simulink model "CAMFC2_Quad_New_02_Payload_01"  (R2018b)
settings: Solver=ode45  StartTime=0.0  StopTime=200  RelTol=1e-3  EnableMultiTasking=on
InitFcn:
  | constant_CAMFC2_Quad_New_02_Payload_01
values from neighbouring files (symbols this model uses):
  alpha = 0.01    [constant_CAMFC2_Quad_New_02_Payload_01.m]
  AN = [     0 1 0 0 ... (first row only)    [constant_CAMFC2_Quad_New_02_Payload_01.m]
  B = 1e0*eye(n)    [Simple_2Quad_payload_03_const.m]    (also in constant_CAMFC2_Quad_New_02_Payload_01.m = eye(n); test01.m = [eye(3) eye(3) eye(3) eye(3))
  B_pseudo_inverse = ((B'*B)^(-1))*B'    [constant_CAMFC2_Quad_New_02_Payload_01.m]
  BBT_inv = ((B'*B)^(-1))*B'    [Simple_2Quad_payload_03_const.m]    (also in Simple_4Quad_payload_04_const.m = ((BR'*BR)^(-1))*BR'; Simple_4Quad_payload_05_const.m = ((BR'*BR)^(-1))*BR'; Simple_4Quad_payload_06_const.m = ((BR'*BR)^(-1))*BR'; Simple_4Quad_payload_07_const.m = ((BR'*BR)^(-1))*BR')
  Beta = 0.1    [constant_CAMFC2_Quad_New_02_Payload_01.m]
  BN = [     1 0 0 0 ... (first row only)    [constant_CAMFC2_Quad_New_02_Payload_01.m]
  epsilon_struct = struct('data',epsilon_InitVal)    [constant_CAMFC2_Quad_New_02_Payload_01.m]
  gama1 = 1e+3*diag([1e-6*ones(n0,1);1e-0*ones(n0,1)])    [constant_CAMFC2_Quad_New_02_Payload_01.m]
  gama2 = 1e-1*diag([1e-6*ones(n0,1);1e-0*ones(n0,1)])    [constant_CAMFC2_Quad_New_02_Payload_01.m]
  gamma_0 = 1e-0*diag([1e-3;1e-0])    [Simple_2Quad_payload_03_const.m]    (also in Simple_4Quad_payload_04_const.m = 1e-0*diag([1e-6*ones(3,1);1e-0*ones(3,1)]); Simple_4Quad_payload_05_const.m = 1e-1*diag([1e-6*ones(3,1);1e-0*ones(3,1)]); Simple_4Quad_payload_06_const.m = 1e-0*diag([1e-6*ones(3,1);1e-0*ones(3,1)]); Simple_4Quad_payload_07_const.m = 1e-0*diag([1e-6*ones(3,1);1e-0*ones(3,1)]))
  gamma_1 = 1e+2*diag([1e-3;1e-0])    [Simple_2Quad_payload_03_const.m]    (also in Simple_4Quad_payload_04_const.m = 1e+2*diag([1e-6*ones(3,1);1e-0*ones(3,1)]); Simple_4Quad_payload_05_const.m = 1e+2*diag([1e-6*ones(3,1);1e-0*ones(3,1)]); Simple_4Quad_payload_06_const.m = 1e+3*diag([1e-6*ones(3,1);1e-0*ones(3,1)]); Simple_4Quad_payload_07_const.m = 1e+3*diag([1e-6*ones(3,1);1e-0*ones(3,1)]))
  ge = 9.81    [Simple_4Quad_payload_03_const.m]    (also in constant_CAMFC2_Quad_New_02_Payload_01.m)
  H = L + BN    [constant_CAMFC2_Quad_New_02_Payload_01.m]
  J = 1.2416e-3 * diag([1 1 2],0)    [constant_CAMFC2_Quad_New_02_Payload_01.m]
  K = 1e+1*eye(n)    [constant_CAMFC2_Quad_New_02_Payload_01.m]
  k1 = 1    [Simple_2Quad_payload_03_const.m]    (also in Simple_4Quad_payload_04_const.m; Simple_4Quad_payload_05_const.m; Simple_4Quad_payload_06_const.m; Simple_4Quad_payload_07_const.m)
  k2 = 0.1    [Simple_2Quad_payload_03_const.m]    (also in Simple_4Quad_payload_04_const.m; Simple_4Quad_payload_05_const.m; Simple_4Quad_payload_06_const.m; Simple_4Quad_payload_07_const.m)
  Ka = 0.01    [Simple_4Quad_payload_03_const.m]    (also in constant_CAMFC2_Quad_New_02_Payload_01.m)
  Kd = 0.01    [Simple_4Quad_payload_03_const.m]    (also in constant_CAMFC2_Quad_New_02_Payload_01.m)
  Kf = 1.0e-5    (= 1e-05)    [Simple_4Quad_payload_03_const.m]    (also in constant_CAMFC2_Quad_New_02_Payload_01.m)
  Kt = 0.0435 * Kf    (= 4.35e-07)    [Simple_4Quad_payload_03_const.m]    (also in constant_CAMFC2_Quad_New_02_Payload_01.m = 1e-07)
  Lq = 0.45    [Simple_4Quad_payload_03_const.m]    (also in constant_CAMFC2_Quad_New_02_Payload_01.m = 0.2)
  m = 1.5    [Colab_4Quad_model_01_const.m]    (also in Colab_4Quad_model_02_const.m; Simple_2Quad_payload_04_const.m = 1; Simple_4Quad_payload_01_const.m = 1; Simple_4Quad_payload_02_const.m = 1)
  M = 1.0    (= 1)    [Colab_4Quad_model_01_const.m]    (also in Colab_4Quad_model_02_const.m; Simple_2Quad_payload_01_const.m; Simple_2Quad_payload_02_const.m; Simple_2Quad_payload_03_const.m)
  mp = 10    [constant_CAMFC2_Quad_New_02_Payload_01.m]
  N = 4    [constant_CAMFC2_Quad_New_02_Payload_01.m]
  n = 2    [Simple_2Quad_payload_03_const.m]    (also in Simple_4Quad_payload_03_const.m = 6; Simple_4Quad_payload_04_const.m = 6; Simple_4Quad_payload_05_const.m = 6; Simple_4Quad_payload_06_const.m = 6)
  n0 = 3    [constant_CAMFC2_Quad_New_02_Payload_01.m]
  np = 3    [Simple_4Quad_payload_10_const.m]    (also in Simple_4Quad_payload_11_const.m; Simple_4Quad_payload_12_const.m; constant_CAMFC2_Quad_New_02_Payload_01.m = 6)
  Observer_Gain = 10    [constant_CAMFC2_Quad_New_02_Payload_01.m]
  Observer_Gain1 = 10    [constant_CAMFC2_Quad_New_02_Payload_01.m]
  P_struct = struct('data',P_InitVal)    [constant_CAMFC2_Quad_New_02_Payload_01.m]
  Q = 1e-1*eye(n)    [Simple_2Quad_payload_03_const.m]    (also in constant_CAMFC2_Quad_New_02_Payload_01.m = 1e+1*eye(n))
  QR = 1e-0*eye(n)    [Simple_4Quad_payload_04_const.m]    (also in Simple_4Quad_payload_05_const.m = 1e-1*eye(n); Simple_4Quad_payload_06_const.m; Simple_4Quad_payload_07_const.m; Simple_4Quad_payload_08_const.m)
  R = 1e+0*eye(n)    [Simple_2Quad_payload_03_const.m]    (also in Simple_4Quad_payload_04_const.m = 1e+0*eye(m); Simple_4Quad_payload_05_const.m = 1e+0*eye(m); Simple_4Quad_payload_06_const.m; Simple_4Quad_payload_07_const.m)
  r_formX = 1.0    (= 1)    [constant_CAMFC2_Quad_New_02_Payload_01.m]
  r_formY = 1.0    (= 1)    [constant_CAMFC2_Quad_New_02_Payload_01.m]
  r_formZ = 1.0    (= 1)    [constant_CAMFC2_Quad_New_02_Payload_01.m]
  rho1 = 1e-0    (= 1)    [constant_CAMFC2_Quad_New_02_Payload_01.m]
  rho2 = 1e-1    (= 0.1)    [constant_CAMFC2_Quad_New_02_Payload_01.m]
  rho_0 = 1e-0    (= 1)    [Simple_2Quad_payload_03_const.m]    (also in Simple_4Quad_payload_04_const.m; Simple_4Quad_payload_05_const.m = 0.1; Simple_4Quad_payload_06_const.m; Simple_4Quad_payload_07_const.m)
  rho_1 = 1e-0    (= 1)    [Simple_2Quad_payload_03_const.m]    (also in Simple_4Quad_payload_04_const.m; Simple_4Quad_payload_05_const.m; Simple_4Quad_payload_06_const.m; Simple_4Quad_payload_07_const.m)
  T_struct = struct('data',T_InitVal)    [constant_CAMFC2_Quad_New_02_Payload_01.m]
  U_dot0_M = U_dot0_m*ones(n0,1)    [constant_CAMFC2_Quad_New_02_Payload_01.m]
  Upsilon_M = Upsilon_m*ones(n0,1)    [constant_CAMFC2_Quad_New_02_Payload_01.m]
  X_M = X_m*ones(n0,1)    [constant_CAMFC2_Quad_New_02_Payload_01.m]
(part 2 of 3)

== system CAMFC2_Quad_New_02_Payload_01/Data Bus /Reference Trajectory/Differentiator0 ==
  x_d : Inport
  Integrator : Integrator  InitialCondition=zeros(n0,1)
  Integrator1 : Integrator  InitialCondition=zeros(n0,1)
  Sliding differentiator : MATLAB Function  TreatAsAtomicUnit=on
  Sliding differentiator1 : MATLAB Function  TreatAsAtomicUnit=on
  Sum : Sum  Inputs=|-+
  Dx_d : Outport
  wires:
  Sliding differentiator/1(u) -> Integrator1/1, Dx_d/1
  Sliding differentiator1/1(Du1) -> Integrator/1
  Integrator/1 -> Sliding differentiator/1(u1)
  x_d/1 -> Sum/1
  Sum/1 -> Sliding differentiator/2(e), Sliding differentiator1/1(e)
  Integrator1/1 -> Sum/2

== system CAMFC2_Quad_New_02_Payload_01/Data Bus /Reference Trajectory/Subsystem ==
  Clock1 : Clock
  Desired Position4 : Constant  Value=0  VectorParams1D=off
  From Workspace : FromWorkspace  VariableName=RECT_X  SampleTime=0
  From Workspace1 : FromWorkspace  VariableName=RECT_Y  SampleTime=0
  From Workspace3 : FromWorkspace  VariableName=RECT_Z  SampleTime=0
  Gain : Gain
  Gain1 : Gain
  Gain2 : Gain
  Scope2 : Scope  NumInputPorts=3
  Switch : Switch  Criteria=u2 > Threshold  Threshold=10
  Transfer Fcn1 : TransferFcn  Numerator=[Beta]  Denominator=[1 Beta]
  Transfer Fcn2 : TransferFcn  Numerator=[Beta]  Denominator=[1 Beta]
  Transfer Fcn3 : TransferFcn  Numerator=[Beta]  Denominator=[1 Beta]
  Xd : Outport
  Yd : Outport  Port=2
  Zd : Outport  Port=3
  wires:
  Clock1/1 -> Switch/2
  Switch/1 -> Transfer Fcn1/1
  From Workspace3/1 -> Gain2/1
  Desired Position4/1 -> Switch/3
  Transfer Fcn1/1 -> Zd/1, Scope2/3
  Transfer Fcn2/1 -> Yd/1, Scope2/2
  Transfer Fcn3/1 -> Xd/1, Scope2/1
  Gain/1 -> Transfer Fcn3/1
  Gain1/1 -> Transfer Fcn2/1
  Gain2/1 -> Switch/1

== system CAMFC2_Quad_New_02_Payload_01/Data Bus /Rotational Log/For matrix Plot ==
  P : Inport
  MATLAB Function : MATLAB Function  TreatAsAtomicUnit=on
  To Workspace : ToWorkspace  VariableName=P1_R  SaveFormat=Structure With Time  SampleTime=-1
  wires:
  MATLAB Function/1(y) -> To Workspace/1
  P/1 -> MATLAB Function/1(u)

== system CAMFC2_Quad_New_02_Payload_01/Data Bus /Rotational Log/For matrix Plot1 ==
  P : Inport
  MATLAB Function : MATLAB Function  TreatAsAtomicUnit=on
  To Workspace : ToWorkspace  VariableName=P2_R  SaveFormat=Structure With Time  SampleTime=-1
  wires:
  P/1 -> MATLAB Function/1(u)
  MATLAB Function/1(y) -> To Workspace/1

== system CAMFC2_Quad_New_02_Payload_01/Data Bus /Rotational Log/For matrix Plot2 ==
  P : Inport
  MATLAB Function : MATLAB Function  TreatAsAtomicUnit=on
  To Workspace : ToWorkspace  VariableName=P3_R  SaveFormat=Structure With Time  SampleTime=-1
  wires:
  P/1 -> MATLAB Function/1(u)
  MATLAB Function/1(y) -> To Workspace/1

== system CAMFC2_Quad_New_02_Payload_01/Data Bus /Rotational Log/For matrix Plot3 ==
  P : Inport
  MATLAB Function : MATLAB Function  TreatAsAtomicUnit=on
  To Workspace : ToWorkspace  VariableName=P4_R  SaveFormat=Structure With Time  SampleTime=-1
  wires:
  MATLAB Function/1(y) -> To Workspace/1
  P/1 -> MATLAB Function/1(u)

== system CAMFC2_Quad_New_02_Payload_01/Data Bus /Rotational Log/For matrix Plot4 ==
  A_hat : Inport
  MATLAB Function : MATLAB Function  TreatAsAtomicUnit=on
  To Workspace : ToWorkspace  VariableName=A_hat1_R  SaveFormat=Structure With Time  SampleTime=-1
  wires:
  A_hat/1 -> MATLAB Function/1(u)
  MATLAB Function/1(y) -> To Workspace/1

== system CAMFC2_Quad_New_02_Payload_01/Data Bus /Rotational Log/For matrix Plot5 ==
  A_hat : Inport
  MATLAB Function : MATLAB Function  TreatAsAtomicUnit=on
  To Workspace : ToWorkspace  VariableName=A_hat2_R  SaveFormat=Structure With Time  SampleTime=-1
  wires:
  MATLAB Function/1(y) -> To Workspace/1
  A_hat/1 -> MATLAB Function/1(u)

== system CAMFC2_Quad_New_02_Payload_01/Data Bus /Rotational Log/For matrix Plot6 ==
  A_hat : Inport
  MATLAB Function : MATLAB Function  TreatAsAtomicUnit=on
  To Workspace : ToWorkspace  VariableName=A_hat3_R  SaveFormat=Structure With Time  SampleTime=-1
  wires:
  A_hat/1 -> MATLAB Function/1(u)
  MATLAB Function/1(y) -> To Workspace/1

== system CAMFC2_Quad_New_02_Payload_01/Data Bus /Rotational Log/For matrix Plot7 ==
  A_hat : Inport
  MATLAB Function : MATLAB Function  TreatAsAtomicUnit=on
  To Workspace : ToWorkspace  VariableName=A_hat4_R  SaveFormat=Structure With Time  SampleTime=-1
  wires:
  MATLAB Function/1(y) -> To Workspace/1
  A_hat/1 -> MATLAB Function/1(u)

== system CAMFC2_Quad_New_02_Payload_01/Data Bus /Translational Log/For matrix Plot ==
  P : Inport
  MATLAB Function : MATLAB Function  TreatAsAtomicUnit=on
  To Workspace : ToWorkspace  VariableName=P1_T  SaveFormat=Structure With Time  SampleTime=-1
  wires:
  P/1 -> MATLAB Function/1(u)
  MATLAB Function/1(y) -> To Workspace/1

== system CAMFC2_Quad_New_02_Payload_01/Data Bus /Translational Log/For matrix Plot1 ==
  P : Inport
  MATLAB Function : MATLAB Function  TreatAsAtomicUnit=on
  To Workspace : ToWorkspace  VariableName=P2_T  SaveFormat=Structure With Time  SampleTime=-1
  wires:
  MATLAB Function/1(y) -> To Workspace/1
  P/1 -> MATLAB Function/1(u)

== system CAMFC2_Quad_New_02_Payload_01/Data Bus /Translational Log/For matrix Plot2 ==
  P : Inport
  MATLAB Function : MATLAB Function  TreatAsAtomicUnit=on
  To Workspace : ToWorkspace  VariableName=P3_T  SaveFormat=Structure With Time  SampleTime=-1
  wires:
  MATLAB Function/1(y) -> To Workspace/1
  P/1 -> MATLAB Function/1(u)

== system CAMFC2_Quad_New_02_Payload_01/Data Bus /Translational Log/For matrix Plot3 ==
  P : Inport
  MATLAB Function : MATLAB Function  TreatAsAtomicUnit=on
  To Workspace : ToWorkspace  VariableName=P4_T  SaveFormat=Structure With Time  SampleTime=-1
  wires:
  P/1 -> MATLAB Function/1(u)
  MATLAB Function/1(y) -> To Workspace/1

== system CAMFC2_Quad_New_02_Payload_01/Data Bus /Translational Log/For matrix Plot4 ==
  A_hat : Inport
  MATLAB Function : MATLAB Function  TreatAsAtomicUnit=on
  To Workspace : ToWorkspace  VariableName=A_hat1_T  SaveFormat=Structure With Time  SampleTime=-1
  wires:
  MATLAB Function/1(y) -> To Workspace/1
  A_hat/1 -> MATLAB Function/1(u)

== system CAMFC2_Quad_New_02_Payload_01/Data Bus /Translational Log/For matrix Plot5 ==
  A_hat : Inport
  MATLAB Function : MATLAB Function  TreatAsAtomicUnit=on
  To Workspace : ToWorkspace  VariableName=A_hat2_T  SaveFormat=Structure With Time  SampleTime=-1
  wires:
  A_hat/1 -> MATLAB Function/1(u)
  MATLAB Function/1(y) -> To Workspace/1

== system CAMFC2_Quad_New_02_Payload_01/Data Bus /Translational Log/For matrix Plot6 ==
  A_hat : Inport
  MATLAB Function : MATLAB Function  TreatAsAtomicUnit=on
  To Workspace : ToWorkspace  VariableName=A_hat3_T  SaveFormat=Structure With Time  SampleTime=-1
  wires:
  MATLAB Function/1(y) -> To Workspace/1
  A_hat/1 -> MATLAB Function/1(u)

== system CAMFC2_Quad_New_02_Payload_01/Data Bus /Translational Log/For matrix Plot7 ==
  A_hat : Inport
  MATLAB Function : MATLAB Function  TreatAsAtomicUnit=on
  To Workspace : ToWorkspace  VariableName=A_hat4_T  SaveFormat=Structure With Time  SampleTime=-1
  wires:
  A_hat/1 -> MATLAB Function/1(u)
  MATLAB Function/1(y) -> To Workspace/1

== system CAMFC2_Quad_New_02_Payload_01/Agent #1/Controller #1/Cooperative Observers #1/Differentiator2 ==
  x_d : Inport
  Integrator : Integrator  InitialCondition=zeros(N+1,n0)
  Integrator1 : Integrator  InitialCondition=zeros(N+1,n0)
  Sliding differentiator : MATLAB Function  TreatAsAtomicUnit=on
  Sliding differentiator1 : MATLAB Function  TreatAsAtomicUnit=on
  Sum : Sum  Inputs=|-+
  Dx_d : Outport
  wires:
  Sliding differentiator/1(u) -> Integrator1/1, Dx_d/1
  Sliding differentiator1/1(Du1) -> Integrator/1
  Integrator/1 -> Sliding differentiator/1(u1)
  x_d/1 -> Sum/1
  Sum/1 -> Sliding differentiator/2(e), Sliding differentiator1/1(e)
  Integrator1/1 -> Sum/2

== system CAMFC2_Quad_New_02_Payload_01/Agent #1/Controller #1/Rotational/Differentiator ==
  x_d : Inport
  Integrator : Integrator  InitialCondition=zeros(n,1)
  Integrator1 : Integrator  InitialCondition=zeros(n,1)
  Scope : Scope
  Scope1 : Scope
  Sliding differentiator : MATLAB Function  TreatAsAtomicUnit=on
  Sliding differentiator1 : MATLAB Function  TreatAsAtomicUnit=on
  Sum : Sum  Inputs=|-+
  Dx_d : Outport
  wires:
  Sliding differentiator/1(u) -> Scope/1, Integrator1/1, Dx_d/1
  Sliding differentiator1/1(Du1) -> Integrator/1
  Integrator/1 -> Sliding differentiator/1(u1)
  x_d/1 -> Sum/1
  Sum/1 -> Scope1/1, Sliding differentiator/2(e), Sliding differentiator1/1(e)
  Integrator1/1 -> Sum/2

== system CAMFC2_Quad_New_02_Payload_01/Agent #1/Controller #1/Translational #1/Differentiator1 ==
  x_d : Inport
  Integrator : Integrator  InitialCondition=zeros(n0,1)
  Integrator1 : Integrator  InitialCondition=zeros(n0,1)
  Sliding differentiator : MATLAB Function  TreatAsAtomicUnit=on
  Sliding differentiator1 : MATLAB Function  TreatAsAtomicUnit=on
  Sum : Sum  Inputs=|-+
  Dx_d : Outport
  wires:
  Sliding differentiator/1(u) -> Integrator1/1, Dx_d/1
  Sliding differentiator1/1(Du1) -> Integrator/1
  Integrator/1 -> Sliding differentiator/1(u1)
  x_d/1 -> Sum/1
  Sum/1 -> Sliding differentiator/2(e), Sliding differentiator1/1(e)
  Integrator1/1 -> Sum/2

== system CAMFC2_Quad_New_02_Payload_01/Agent #2/Controller #2/Cooperative Observers #2/Differentiator2 ==
  x_d : Inport
  Integrator : Integrator  InitialCondition=zeros(N+1,n0)
  Integrator1 : Integrator  InitialCondition=zeros(N+1,n0)
  Sliding differentiator : MATLAB Function  TreatAsAtomicUnit=on
  Sliding differentiator1 : MATLAB Function  TreatAsAtomicUnit=on
  Sum : Sum  Inputs=|-+
  Dx_d : Outport
  wires:
  Sliding differentiator/1(u) -> Integrator1/1, Dx_d/1
  Sliding differentiator1/1(Du1) -> Integrator/1
  Integrator/1 -> Sliding differentiator/1(u1)
  x_d/1 -> Sum/1
  Sum/1 -> Sliding differentiator/2(e), Sliding differentiator1/1(e)
  Integrator1/1 -> Sum/2

== system CAMFC2_Quad_New_02_Payload_01/Agent #2/Controller #2/Rotational/Differentiator ==
  x_d : Inport
  Integrator : Integrator  InitialCondition=zeros(n,1)
  Integrator1 : Integrator  InitialCondition=zeros(n,1)
  Scope : Scope
  Scope1 : Scope
  Sliding differentiator : MATLAB Function  TreatAsAtomicUnit=on
  Sliding differentiator1 : MATLAB Function  TreatAsAtomicUnit=on
  Sum : Sum  Inputs=|-+
  Dx_d : Outport
  wires:
  Sliding differentiator/1(u) -> Scope/1, Integrator1/1, Dx_d/1
  Sliding differentiator1/1(Du1) -> Integrator/1
  Integrator/1 -> Sliding differentiator/1(u1)
  x_d/1 -> Sum/1
  Sum/1 -> Scope1/1, Sliding differentiator/2(e), Sliding differentiator1/1(e)
  Integrator1/1 -> Sum/2

== system CAMFC2_Quad_New_02_Payload_01/Agent #2/Controller #2/Translational #2/Differentiator1 ==
  x_d : Inport
  Integrator : Integrator  InitialCondition=zeros(n0,1)
  Integrator1 : Integrator  InitialCondition=zeros(n0,1)
  Sliding differentiator : MATLAB Function  TreatAsAtomicUnit=on
  Sliding differentiator1 : MATLAB Function  TreatAsAtomicUnit=on
  Sum : Sum  Inputs=|-+
  Dx_d : Outport
  wires:
  Sliding differentiator/1(u) -> Integrator1/1, Dx_d/1
  Sliding differentiator1/1(Du1) -> Integrator/1
  Integrator/1 -> Sliding differentiator/1(u1)
  x_d/1 -> Sum/1
  Sum/1 -> Sliding differentiator/2(e), Sliding differentiator1/1(e)
  Integrator1/1 -> Sum/2

== system CAMFC2_Quad_New_02_Payload_01/Agent #3/Controller #3/Cooperative Observers #3/Differentiator2 ==
  x_d : Inport
  Integrator : Integrator  InitialCondition=zeros(N+1,n0)
  Integrator1 : Integrator  InitialCondition=zeros(N+1,n0)
  Sliding differentiator : MATLAB Function  TreatAsAtomicUnit=on
  Sliding differentiator1 : MATLAB Function  TreatAsAtomicUnit=on
  Sum : Sum  Inputs=|-+
  Dx_d : Outport
  wires:
  Sliding differentiator/1(u) -> Integrator1/1, Dx_d/1
  Sliding differentiator1/1(Du1) -> Integrator/1
  Integrator/1 -> Sliding differentiator/1(u1)
  x_d/1 -> Sum/1
  Sum/1 -> Sliding differentiator/2(e), Sliding differentiator1/1(e)
  Integrator1/1 -> Sum/2

== system CAMFC2_Quad_New_02_Payload_01/Agent #3/Controller #3/Rotational/Differentiator ==
  x_d : Inport
  Integrator : Integrator  InitialCondition=zeros(n,1)
  Integrator1 : Integrator  InitialCondition=zeros(n,1)
  Scope : Scope
  Scope1 : Scope
  Sliding differentiator : MATLAB Function  TreatAsAtomicUnit=on
  Sliding differentiator1 : MATLAB Function  TreatAsAtomicUnit=on
  Sum : Sum  Inputs=|-+
  Dx_d : Outport
  wires:
  Sliding differentiator/1(u) -> Scope/1, Integrator1/1, Dx_d/1
  Sliding differentiator1/1(Du1) -> Integrator/1
  Integrator/1 -> Sliding differentiator/1(u1)
  x_d/1 -> Sum/1
  Sum/1 -> Scope1/1, Sliding differentiator/2(e), Sliding differentiator1/1(e)
  Integrator1/1 -> Sum/2

== system CAMFC2_Quad_New_02_Payload_01/Agent #3/Controller #3/Translational #3/Differentiator1 ==
  x_d : Inport
  Integrator : Integrator  InitialCondition=zeros(n0,1)
  Integrator1 : Integrator  InitialCondition=zeros(n0,1)
  Sliding differentiator : MATLAB Function  TreatAsAtomicUnit=on
  Sliding differentiator1 : MATLAB Function  TreatAsAtomicUnit=on
  Sum : Sum  Inputs=|-+
  Dx_d : Outport
  wires:
  Sliding differentiator/1(u) -> Integrator1/1, Dx_d/1
  Sliding differentiator1/1(Du1) -> Integrator/1
  Integrator/1 -> Sliding differentiator/1(u1)
  x_d/1 -> Sum/1
  Sum/1 -> Sliding differentiator/2(e), Sliding differentiator1/1(e)
  Integrator1/1 -> Sum/2

== system CAMFC2_Quad_New_02_Payload_01/Agent #4/Controller #4/Cooperative Observers #1/Differentiator2 ==
  x_d : Inport
  Integrator : Integrator  InitialCondition=zeros(N+1,n0)
  Integrator1 : Integrator  InitialCondition=zeros(N+1,n0)
  Sliding differentiator : MATLAB Function  TreatAsAtomicUnit=on
  Sliding differentiator1 : MATLAB Function  TreatAsAtomicUnit=on
  Sum : Sum  Inputs=|-+
  Dx_d : Outport
  wires:
  Sliding differentiator/1(u) -> Integrator1/1, Dx_d/1
  Sliding differentiator1/1(Du1) -> Integrator/1
  Integrator/1 -> Sliding differentiator/1(u1)
  x_d/1 -> Sum/1
  Sum/1 -> Sliding differentiator/2(e), Sliding differentiator1/1(e)
  Integrator1/1 -> Sum/2

== system CAMFC2_Quad_New_02_Payload_01/Agent #4/Controller #4/Rotational/Differentiator ==
  x_d : Inport
  Integrator : Integrator  InitialCondition=zeros(n,1)
  Integrator1 : Integrator  InitialCondition=zeros(n,1)
  Scope : Scope
  Scope1 : Scope
  Sliding differentiator : MATLAB Function  TreatAsAtomicUnit=on
  Sliding differentiator1 : MATLAB Function  TreatAsAtomicUnit=on
  Sum : Sum  Inputs=|-+
  Dx_d : Outport
  wires:
  Sliding differentiator/1(u) -> Scope/1, Integrator1/1, Dx_d/1
  Sliding differentiator1/1(Du1) -> Integrator/1
  Integrator/1 -> Sliding differentiator/1(u1)
  x_d/1 -> Sum/1
  Sum/1 -> Scope1/1, Sliding differentiator/2(e), Sliding differentiator1/1(e)
  Integrator1/1 -> Sum/2

== system CAMFC2_Quad_New_02_Payload_01/Agent #4/Controller #4/Translational #4/Differentiator1 ==
  x_d : Inport
  Integrator : Integrator  InitialCondition=zeros(n0,1)
  Integrator1 : Integrator  InitialCondition=zeros(n0,1)
  Sliding differentiator : MATLAB Function  TreatAsAtomicUnit=on
  Sliding differentiator1 : MATLAB Function  TreatAsAtomicUnit=on
  Sum : Sum  Inputs=|-+
  Dx_d : Outport
  wires:
  Sliding differentiator/1(u) -> Integrator1/1, Dx_d/1
  Sliding differentiator1/1(Du1) -> Integrator/1
  Integrator/1 -> Sliding differentiator/1(u1)
  x_d/1 -> Sum/1
  Sum/1 -> Sliding differentiator/2(e), Sliding differentiator1/1(e)
  Integrator1/1 -> Sum/2

== matlab function CAMFC2_Quad_New_02_Payload_01/Agent #1/Controller #1/Controller to Motors #1 ==
  data: u output; uT input; uR input; RM_1 parameter
function u = fcn(uT,uR,RM_1)

y1 = uR(4);
y2 = uR(5);
y3 = uR(6);

Y = [uT;y1;y2;y3];

u = RM_1*Y;

for i=1:4
    u(i) = sqrt(abs(u(i)));
end

end

== matlab function CAMFC2_Quad_New_02_Payload_01/Agent #2/Controller #2/Controller Interpreter #2 ==
  data: ut_i input; uT_i output; PHI_d_i output
function [uT_i,PHI_d_i] = fcn(ut_i)

%%
f0 = sqrt((ut_i(1)^2)+(ut_i(2)^2)+(ut_i(3)^2));
psi_d = 0;
phi_d = asin( min(max(((sin(psi_d)*ut_i(1) - cos(psi_d)*ut_i(2)) / (f0+1e-3)),-1),1) );
theta_d = atan( (cos(psi_d)*ut_i(1) + sin(psi_d)*ut_i(2)) / (ut_i(3)+1e-3) );
PHI_d_i = [phi_d;theta_d;psi_d]; 
uT_i = f0;

end

== matlab function CAMFC2_Quad_New_02_Payload_01/Payload/Controller /Control law ==
  data: u output; DDp_d input; Dp_d input; e input; Ie input; v input
function u = fcn(DDp_d,Dp_d,e,Ie, v)

k1 = 10;
k2 = 1;
k3 = 1;
u = DDp_d + k2*Dp_d - k2*v + k1*e + k3*Ie;

end

== matlab function CAMFC2_Quad_New_02_Payload_01/Agent #3/Controller #3/Controller Interpreter #3 ==
  data: ut_i input; uT_i output; PHI_d_i output
function [uT_i,PHI_d_i] = fcn(ut_i)

%%
f0 = sqrt((ut_i(1)^2)+(ut_i(2)^2)+(ut_i(3)^2));
psi_d = 0;
phi_d = asin( min(max(((sin(psi_d)*ut_i(1) - cos(psi_d)*ut_i(2)) / (f0+1e-3)),-1),1) );
theta_d = atan( (cos(psi_d)*ut_i(1) + sin(psi_d)*ut_i(2)) / (ut_i(3)+1e-3) );
PHI_d_i = [phi_d;theta_d;psi_d]; 
uT_i = f0;

end

== matlab function CAMFC2_Quad_New_02_Payload_01/Agent #4/Controller #4/Controller Interpreter #4 ==
  data: ut_i input; uT_i output; PHI_d_i output
function [uT_i,PHI_d_i] = fcn(ut_i)

%%
f0 = sqrt((ut_i(1)^2)+(ut_i(2)^2)+(ut_i(3)^2));
psi_d = 0;
phi_d = asin( min(max(((sin(psi_d)*ut_i(1) - cos(psi_d)*ut_i(2)) / (f0+1e-3)),-1),1) );
theta_d = atan( (cos(psi_d)*ut_i(1) + sin(psi_d)*ut_i(2)) / (ut_i(3)+1e-3) );
PHI_d_i = [phi_d;theta_d;psi_d]; 
uT_i = f0;

end

== matlab function CAMFC2_Quad_New_02_Payload_01/Agent #1/Controller #1/Cooperative Observers #1/Differentiator2/Sliding differentiator ==
  data: u output; u1 input; e input; k1 parameter; alpha parameter
function u = fcn(u1,e,k1,alpha)

b=k1;

ABS = abs(e);
SGN = e ./ (ABS + alpha);
u = u1 - b*((ABS.^0.5).*SGN); 

end

== matlab function CAMFC2_Quad_New_02_Payload_01/Agent #1/Controller #1/Cooperative Observers #1/Differentiator2/Sliding differentiator1 ==
  data: Du1 output; e input; k2 parameter; alpha parameter
function Du1 = fcn(e,k2,alpha)

a=k2;

ABS = abs(e);
SGN = e ./ (ABS + alpha);
Du1 = - a*SGN;

end

== matlab function CAMFC2_Quad_New_02_Payload_01/Agent #1/Controller #1/Cooperative Observers #1/Observer T#1 ==
  data: T_struct parameter; T input; DT_i output; epsilon input; epsilon_struct parameter; H parameter; BN parameter; AN parameter; T_i input; Upsilon_M parameter; epsilon_i output; N parameter; n0 parameter; Agent_Num input; Observer_Gain1 parameter; chi input
function [DT_i,epsilon_i] = fcn(T_struct,T,epsilon,epsilon_struct,H,BN,AN,T_i,Upsilon_M,N,n0,Agent_Num,Observer_Gain1, chi)

T_struct(1).data = T.t1;
T_struct(2).data = T.t2;
T_struct(3).data = T.t3;
T_struct(4).data = T.t4;

epsilon_struct(1).data = epsilon.eps1;
epsilon_struct(2).data = epsilon.eps2;
epsilon_struct(3).data = epsilon.eps3;
epsilon_struct(4).data = epsilon.eps4;

epsilon_i = + BN(Agent_Num,Agent_Num)*(T_i - chi);
Sum2 = zeros(N+1,n0);
for i=1:N
    epsilon_i = epsilon_i + ( AN(Agent_Num,i) * (T_i - T_struct(i).data) );  
    Sum2 = Sum2 + ( H(i,Agent_Num) * epsilon_struct(i).data );
end

Sum21 = abs(Sum2) + 0.1;
SGN2 = Sum2./Sum21;

DT_i = -Observer_Gain1*epsilon_i - SGN2*diag(Upsilon_M);

end

== matlab function CAMFC2_Quad_New_02_Payload_01/Agent #1/Controller #1/Cooperative Observers #1/Observer x0_hat#1 ==
  data: x0_hat input; Dx0_hat_i output; x0_tilde input; H parameter; BN parameter; AN parameter; x0_hat_i input; x0 input; X_M parameter; x0_tilde_i output; N parameter; Agent_Num input; Observer_Gain parameter; n0 parameter; alpha parameter
function [Dx0_hat_i,x0_tilde_i] = fcn(x0_hat,x0_tilde,H,BN,AN,x0_hat_i,x0,X_M,N,Agent_Num,Observer_Gain,n0,alpha)

x0_tilde_i = + BN(Agent_Num,Agent_Num)*(x0_hat_i - x0);
Sum2 = zeros(n0,1);
for i=1:N
    x0_tilde_i = x0_tilde_i + ( AN(Agent_Num,i) * (x0_hat_i - x0_hat(((i-1)*n0+1):n0*i)) );  
    Sum2 = Sum2 + ( H(i,Agent_Num) * x0_tilde(((i-1)*n0+1):n0*i) );
end

Sum21 = abs(Sum2) + alpha;
SGN2 = Sum2./Sum21;

Dx0_hat_i = -Observer_Gain*x0_tilde_i - diag(SGN2)*X_M;

end

== matlab function CAMFC2_Quad_New_02_Payload_01/Agent #1/Controller #1/Translational #1/Adaptive Law A_T #1 ==
  data: Agent_Num input; A_hat input; gama2 parameter; rho2 parameter; T_i input; P_i input; DA_hat output; e_i input; H parameter; BN parameter; N parameter; n parameter; n0 parameter; z0 input; x0_hat_inp input; ui input
function DA_hat = fcn(Agent_Num,A_hat,gama2,rho2,T_i,P_i,e_i,H,BN,N,n,n0,z0,x0_hat_inp,ui)

%% 
z0_i = [z0;ui(1:n0)]; 
x0_hat_i = [x0_hat_inp;ui(1:n0)];

%%
vA_hat = diag(A_hat);

Sum = zeros(n,1);
for i=2:(N+1)
    Sum = Sum + ( H(Agent_Num,(i-1)) * ( (2*x0_hat_i) - (2*[T_i(1,:)';zeros(n0,1)]) + ([T_i(i,:)';zeros(n0,1)]) ) );
end
Sum(1:n0) = Sum(1:n0) + ( BN(Agent_Num,Agent_Num)*z0_i(1:n0) ) - e_i(1:n0);
Sum(n0+1:n) = Sum(n0+1:n) + ( 1*z0_i(n0+1:n) ) - e_i(n0+1:n);
    
DvA_hat = -gama2*diag(Sum)*P_i * e_i - (rho2*gama2*vA_hat);

DA_hat = diag(DvA_hat);

end

== matlab function CAMFC2_Quad_New_02_Payload_01/Payload/Plant/MATLAB Function ==
  data: X input; U input; DX output; ge parameter; mp parameter
function DX = fcn(X,U,ge, mp)

V = X(4:6);
DX = [V;(U-[0;0;(mp*ge)])];

end

== matlab function CAMFC2_Quad_New_02_Payload_01/Agent #1/Controller #1/Cooperative Observers #1/Observer q#1 ==
  data: q input; Dq_i output; tau input; H parameter; BN parameter; AN parameter; q_i input; u0 input; U_dot0_M parameter; tau_i output; N parameter; Agent_Num input; Observer_Gain parameter; n0 parameter; alpha parameter
function [Dq_i,tau_i] = fcn(q,tau,H,BN,AN,q_i,u0,U_dot0_M,N,Agent_Num,Observer_Gain,n0,alpha)

tau_i = + BN(Agent_Num,Agent_Num)*(q_i - u0);
Sum2 = zeros(n0,1);
for i=1:N
    tau_i = tau_i + ( AN(Agent_Num,i) * (q_i - q(((i-1)*n0+1):n0*i)) );  
    Sum2 = Sum2 + ( H(i,Agent_Num) * tau(((i-1)*n0+1):n0*i) );
end

Sum21 = abs(Sum2) + alpha;
SGN2 = Sum2./Sum21;

Dq_i = -Observer_Gain*tau_i - diag(SGN2)*U_dot0_M;

end

== matlab function CAMFC2_Quad_New_02_Payload_01/Agent #1/Controller #1/Translational #1/Adaptive Law g_T #1 ==
  data: Agent_Num input; g_hat input; gama1 parameter; rho1 parameter; P input; P_struct parameter; Dg_hat output; e input; H parameter; N parameter; n parameter
function Dg_hat = fcn(Agent_Num,g_hat,gama1,rho1,P,P_struct,e,H,N,n)

P_struct(1).data = P.p1;
P_struct(2).data = P.p2;
P_struct(3).data = P.p3;
P_struct(4).data = P.p4;

Sum = zeros(n,1);
for i=1:N  
    Sum = Sum + (H(i,Agent_Num) * P_struct(i).data * e((i-1)*n+1:(i*n),1)); %Adaptive law
end
    
Dg_hat = -gama1*Sum - (rho1*gama1*g_hat);

end

== matlab function CAMFC2_Quad_New_02_Payload_01/Agent #1/Plant #1/MATLAB Function ==
  data: X input; U input; t input; DX output; Kf parameter; Kt parameter; Kd parameter; Ka parameter; M parameter; J parameter; Lq parameter; ge parameter
function DX = fcn(X,U,t,Kf,Kt,Kd,Ka,M,J,Lq,ge)

phi = X(4);
theta = X(5);
psi = X(6);

Rq = [cos(psi)*cos(theta) -sin(psi)*cos(phi)+cos(psi)*sin(theta)*sin(phi) sin(psi)*sin(phi)+cos(psi)*sin(theta)*cos(phi);
    sin(psi)*cos(theta) cos(psi)*cos(phi)+sin(psi)*sin(theta)*sin(phi) -cos(psi)*sin(phi)+sin(psi)*sin(theta)*cos(phi);
    -sin(theta) cos(theta)*sin(phi) cos(theta)*cos(phi)]; 

R_omega = [1 0 -sin(theta);
    0 cos(phi) cos(theta)*sin(phi);
    0 -sin(phi) cos(theta)*cos(phi)];

EXT_PRD = External_Product3(X(10:12),(J*X(10:12)));

F1 = Kf * U(1)^2;
F2 = Kf * U(2)^2;
F3 = Kf * U(3)^2;
F4 = Kf * U(4)^2;
  
FT = F1 + F2 + F3 + F4;
 
T1 = Kt * U(1)^2;
T2 = Kt * U(2)^2;
T3 = Kt * U(3)^2;
T4 = Kt * U(4)^2;
 
TT1 = Lq*(F3-F1);
TT2 = Lq*(F4-F2);
TT3 = (T1-T2+T3-T4);

FTT = Rq * [0;0;FT];
FTx = FTT(1);
FTy = FTT(2);
FTz = FTT(3);

DP = X(7:9);
DPHI = (R_omega)^(-1) * X(10:12); 
Dv = (1/M)*([FTx;FTy;FTz] - Kd*X(7:9) - M*[0;0;ge]) + Rq*(0.1*sin(1*t))*[0;0;1]; 
Dw = (J^(-1))*([TT1;TT2;TT3] - Ka*X(10:12) - EXT_PRD) + (1*sin(1*t)*[1;1;1]);

DX = [DP;DPHI;Dv;Dw];

end

== matlab function CAMFC2_Quad_New_02_Payload_01/Agent #1/Controller #1/Translational #1/DRE_T ==
  data: P input; A_hat input; B parameter; R parameter; DP output; Q parameter
function DP = fcn(P,A_hat,B,R,Q)

DP = 2*A_hat*P + 2*P*A_hat' - P*B*R*B'*P + 2*Q;

end

== matlab function CAMFC2_Quad_New_02_Payload_01/Agent #3/Controller #3/Controller to Motors #3 ==
  data: u output; uT input; uR input; RM_1 parameter
function u = fcn(uT,uR,RM_1)

y1 = uR(4);
y2 = uR(5);
y3 = uR(6);

Y = [uT;y1;y2;y3];

u = RM_1*Y;

for i=1:4
    u(i) = sqrt(abs(u(i)));
end

end

== matlab function CAMFC2_Quad_New_02_Payload_01/Agent #1/Controller #1/Translational #1/Differentiator1/Sliding differentiator ==
  data: u output; u1 input; e input; k1 parameter; alpha parameter
function u = fcn(u1,e,k1,alpha)

b=k1;

ABS = abs(e);
SGN = e ./ (ABS + alpha);
u = u1 - b*((ABS.^0.5).*SGN); 

end

== matlab function CAMFC2_Quad_New_02_Payload_01/Agent #1/Controller #1/Translational #1/Differentiator1/Sliding differentiator1 ==
  data: Du1 output; e input; k2 parameter; alpha parameter
function Du1 = fcn(e,k2,alpha)

a=k2;

ABS = abs(e);
SGN = e ./ (ABS + alpha);
Du1 = - a*SGN;

end

== matlab function CAMFC2_Quad_New_02_Payload_01/Agent #1/Controller #1/Translational #1/Main Controller_T #1 ==
  data: n parameter; n0 parameter; U output; R parameter; Q parameter; P_i input; e_i input; K parameter; Zeta_i input; BN parameter; A_hat_i input; u0 input; z0 input; DT_i input; T_i input; H parameter; q_i input; Agent_Num input; B_pseudo_inverse parameter; ui input; x0_hat_inp input; g_hat_i input; D_ui1 input
function U = fcn(n,n0,R,Q,P_i,e_i,K,Zeta_i,BN,A_hat_i,u0,z0,DT_i,T_i,H,q_i,Agent_Num,B_pseudo_inverse,ui,x0_hat_inp, g_hat_i, D_ui1)

D_eta_0 = [DT_i(1,:)';zeros(n0,1)];

%% 
z0_i = [z0;ui(1:n0)];
x0_hat_i = [x0_hat_inp;ui(1:n0)];
u0_i = [u0;D_ui1];

%%

S_H = sum(H(Agent_Num,:)) - H(Agent_Num,Agent_Num);
U4 = - S_H * ([q_i;u0_i(n0+1:n)] - [DT_i(1,:)';zeros(n0,1)] - (A_hat_i * (x0_hat_i - [T_i(1,:)';zeros(n0,1)])));
U1 = 1/2 * R * P_i * e_i; %Consensus Error
U5 = ( A_hat_i * ( H(Agent_Num,Agent_Num)*(2*x0_hat_i - 2*[T_i(1,:)';zeros(n0,1)] + [T_i(Agent_Num+1,:)';zeros(n0,1)]) ) ) - e_i;
U5(1:n0) = U5(1:n0) + ( BN(Agent_Num,Agent_Num) * z0_i(1:n0) );
U5(n0+1:n) = U5(n0+1:n) + ( 1 * z0_i(n0+1:n) );
U2 = - g_hat_i; %nonlinear compensation 
U3 = + [DT_i(Agent_Num+1,:)';zeros(n0,1)]; %Derivative of Formation parameters  
U6 = zeros(n,1);
U6(1:n0) = - BN(Agent_Num,Agent_Num)*( D_eta_0(1:n0) - u0_i(1:n0) ); %Connection to the leader
U6(n0+1:n) = - 1 * ( D_eta_0(n0+1:n) - u0_i(n0+1:n) );
U7 = K * Zeta_i; %Consensus time-integral
U8 = (2*Q - 3/4*R*P_i)*e_i;

U_input = U1 + U2 + U3 + U4 + U5 + U6 + U7 + U8;

U = B_pseudo_inverse * U_input / H(Agent_Num,Agent_Num);

end

== matlab function CAMFC2_Quad_New_02_Payload_01/Agent #1/Controller #1/Translational #1/Module to compute Consensus Error_T #1 ==
  data: T_i input; x input; x0 input; ep output; AN parameter; BN parameter; N parameter; n parameter; n0 parameter; Agent_Num input; ui input
function ep = fcn(T_i,x,x0,AN,BN,N,n,n0,Agent_Num,ui)

Diff_Star_to0 = (T_i((Agent_Num+1),:))';
Diff_Star_to_Other = (eye(n0) * Diff_Star_to0 * ones(1,N))' - T_i(2:N+1,:);
Diff_Star_to_Other = Diff_Star_to_Other';

xp = zeros(n,N);
for i=1:N
    xp(1:n,i) = [x((i-1)*(2*n)+1:(i-1)*(2*n)+n0);x((i-1)*(2*n)+(2*n0)+1:(i-1)*(2*n)+(2*n0)+n0)];
end

%%
xp_own = zeros(n,1);
xp_own(1:n,1) = xp(1:n,Agent_Num);

xp0 = [x0;ui(1:n0)];

xp_other = zeros(n,N);
ep = zeros(n,1);
ep(1:n0,1) = ep(1:n0,1) + ( BN(Agent_Num,Agent_Num)*(-(xp_own(1:n0)-xp0(1:n0))+Diff_Star_to0) );
ep(n0+1:n,1) = ep(n0+1:n,1) + ( 1*(-(xp_own(n0+1:n)-xp0(n0+1:n))) );

for i=1:N        
    xp_other(1:n,i) = xp(1:n,i);
    ep(1:n0,1) = ep(1:n0,1) + AN(Agent_Num,i)*(-(xp_own(1:n0)-xp_other(1:n0,i))+Diff_Star_to_Other(:,i));
    ep(n0+1:n,1) = ep(n0+1:n,1) + AN(Agent_Num,i)*(-(xp_own(n0+1:n)-xp_other(n0+1:n,i)));
end

end

== matlab function CAMFC2_Quad_New_02_Payload_01/Agent #3/Controller #3/Cooperative Observers #3/Differentiator2/Sliding differentiator ==
  data: u output; u1 input; e input; k1 parameter; alpha parameter
function u = fcn(u1,e,k1,alpha)

b=k1;

ABS = abs(e);
SGN = e ./ (ABS + alpha);
u = u1 - b*((ABS.^0.5).*SGN); 

end

== matlab function CAMFC2_Quad_New_02_Payload_01/Agent #3/Controller #3/Rotational/CARE ==
  data: P input; a_hat input; B parameter; R parameter; DP output; QR parameter
function DP = fcn(P,a_hat,B,R,QR)

DP = a_hat*P + P*a_hat' - P*B*R*B'*P + 2*QR;

end

== matlab function CAMFC2_Quad_New_02_Payload_01/Agent #3/Controller #3/Rotational/Differentiator/Sliding differentiator ==
  data: u output; u1 input; e input; n parameter; k1 parameter
function u = fcn(u1,e,n,k1)

b=k1;

ABS = zeros(n,1);
for i=1:n
    if e(i)>0
        ABS(i) = e(i);
    else
        ABS(i) = -e(i);
    end
end
SGN = e ./ (ABS + 0.01);

u = u1 - b*(ABS.^0.5).*SGN;

end

== matlab function CAMFC2_Quad_New_02_Payload_01/Agent #3/Controller #3/Rotational/Differentiator/Sliding differentiator1 ==
  data: Du1 output; e input; n parameter; k2 parameter
function Du1 = fcn(e,n,k2)

a=k2;

ABS = zeros(n,1);
for i=1:n
    if e(i)>0
        ABS(i) = e(i);
    else
        ABS(i) = -e(i);
    end
end
SGN = e ./ (ABS + 0.01);

Du1 = - a*SGN;

end

== matlab function CAMFC2_Quad_New_02_Payload_01/Agent #3/Controller #3/Rotational/g-Estimator ==
  data: sigma input; g_hat input; P input; rho_1 parameter; gamma_1 parameter; Dg_hat output
function Dg_hat = fcn(sigma,g_hat,P,rho_1,gamma_1)

Dg_hat = - gamma_1 * P * sigma - rho_1 * gamma_1 * g_hat;

end

== matlab function CAMFC2_Quad_New_02_Payload_01/Agent #3/Controller #3/Rotational/g-Estimator1 ==
  data: sigma input; x input; P input; rho_0 parameter; gamma_0 parameter; Da_hat output; a_hat input
function Da_hat = fcn(sigma,x,P,rho_0,gamma_0,a_hat)

DVa_hat = - gamma_0 * P * diag(sigma) * (x - sigma) - rho_0 * gamma_0 * diag(a_hat);

Da_hat = diag(DVa_hat);

end

== matlab function CAMFC2_Quad_New_02_Payload_01/Agent #3/Controller #3/Rotational/main ==
  data: sigma input; zeta input; u output; Dy_d input; R parameter; P input; a_hat input; B parameter; g_hat input; x input; QR parameter; BBT_inv parameter; n parameter
function u = fcn(sigma,zeta,Dy_d,R,P,a_hat,B,g_hat,x,QR,BBT_inv,n)

u1 = (1/2) * R * B' * P * sigma;
u2 = BBT_inv * (Dy_d - a_hat*x + (eye(n) + 2*(((P)^(-1)*QR)) + a_hat)*sigma - g_hat - zeta) - (3/4) * R * B' * P * sigma;

u = u1 + u2;

end

== matlab function CAMFC2_Quad_New_02_Payload_01/Agent #2/Plant #2/MATLAB Function ==
  data: X input; U input; t input; DX output; Kf parameter; Kt parameter; Kd parameter; Ka parameter; M parameter; J parameter; Lq parameter; ge parameter
function DX = fcn(X,U,t,Kf,Kt,Kd,Ka,M,J,Lq,ge)

phi = X(4);
theta = X(5);
psi = X(6);

Rq = [cos(psi)*cos(theta) -sin(psi)*cos(phi)+cos(psi)*sin(theta)*sin(phi) sin(psi)*sin(phi)+cos(psi)*sin(theta)*cos(phi);
    sin(psi)*cos(theta) cos(psi)*cos(phi)+sin(psi)*sin(theta)*sin(phi) -cos(psi)*sin(phi)+sin(psi)*sin(theta)*cos(phi);
    -sin(theta) cos(theta)*sin(phi) cos(theta)*cos(phi)]; 

R_omega = [1 0 -sin(theta);
    0 cos(phi) cos(theta)*sin(phi);
    0 -sin(phi) cos(theta)*cos(phi)];

EXT_PRD = External_Product3(X(10:12),(J*X(10:12)));

F1 = Kf * U(1)^2;
F2 = Kf * U(2)^2;
F3 = Kf * U(3)^2;
F4 = Kf * U(4)^2;
  
FT = F1 + F2 + F3 + F4;
 
T1 = Kt * U(1)^2;
T2 = Kt * U(2)^2;
T3 = Kt * U(3)^2;
T4 = Kt * U(4)^2;
 
TT1 = Lq*(F3-F1);
TT2 = Lq*(F4-F2);
TT3 = (T1-T2+T3-T4);

FTT = Rq * [0;0;FT];
FTx = FTT(1);
FTy = FTT(2);
FTz = FTT(3);

DP = X(7:9);
DPHI = (R_omega)^(-1) * X(10:12); 
Dv = (1/M)*([FTx;FTy;FTz] - Kd*X(7:9) - M*[0;0;ge]) + Rq*(0.1*sin(1*t))*[0;0;1]; 
Dw = (J^(-1))*([TT1;TT2;TT3] - Ka*X(10:12) - EXT_PRD) + (1*sin(1*t)*[1;1;1]);

DX = [DP;DPHI;Dv;Dw];

end

== matlab function CAMFC2_Quad_New_02_Payload_01/Agent #3/Controller #3/Rotational/variable change ==
  data: X input; Xd input; x_mod output; u input; xd_mod output; e_mod output
function [x_mod,xd_mod,e_mod] = fcn(X,Xd,u)

x_mod = [X(4:6);X(10:12)];

xd_mod = [Xd;u(1:3)];

e_mod = xd_mod - x_mod;


end

== matlab function CAMFC2_Quad_New_02_Payload_01/Agent #4/Controller #4/Rotational/CARE ==
  data: P input; a_hat input; B parameter; R parameter; DP output; QR parameter
function DP = fcn(P,a_hat,B,R,QR)

DP = a_hat*P + P*a_hat' - P*B*R*B'*P + 2*QR;

end

== matlab function CAMFC2_Quad_New_02_Payload_01/Agent #4/Controller #4/Rotational/Differentiator/Sliding differentiator ==
  data: u output; u1 input; e input; n parameter; k1 parameter
function u = fcn(u1,e,n,k1)

b=k1;

ABS = zeros(n,1);
for i=1:n
    if e(i)>0
        ABS(i) = e(i);
    else
        ABS(i) = -e(i);
    end
end
SGN = e ./ (ABS + 0.01);

u = u1 - b*(ABS.^0.5).*SGN;

end

== matlab function CAMFC2_Quad_New_02_Payload_01/Agent #3/Controller #3/Cooperative Observers #3/Differentiator2/Sliding differentiator1 ==
  data: Du1 output; e input; k2 parameter; alpha parameter
function Du1 = fcn(e,k2,alpha)

a=k2;

ABS = abs(e);
SGN = e ./ (ABS + alpha);
Du1 = - a*SGN;

end

== matlab function CAMFC2_Quad_New_02_Payload_01/Agent #3/Controller #3/Cooperative Observers #3/Observer T#3 ==
  data: T_struct parameter; T input; DT_i output; epsilon input; epsilon_struct parameter; H parameter; BN parameter; AN parameter; T_i input; Upsilon_M parameter; epsilon_i output; N parameter; n0 parameter; Agent_Num input; Observer_Gain1 parameter; chi input
function [DT_i,epsilon_i] = fcn(T_struct,T,epsilon,epsilon_struct,H,BN,AN,T_i,Upsilon_M,N,n0,Agent_Num,Observer_Gain1, chi)

T_struct(1).data = T.t1;
T_struct(2).data = T.t2;
T_struct(3).data = T.t3;
T_struct(4).data = T.t4;

epsilon_struct(1).data = epsilon.eps1;
epsilon_struct(2).data = epsilon.eps2;
epsilon_struct(3).data = epsilon.eps3;
epsilon_struct(4).data = epsilon.eps4;

epsilon_i = + BN(Agent_Num,Agent_Num)*(T_i - chi);
Sum2 = zeros(N+1,n0);
for i=1:N
    epsilon_i = epsilon_i + ( AN(Agent_Num,i) * (T_i - T_struct(i).data) );  
    Sum2 = Sum2 + ( H(i,Agent_Num) * epsilon_struct(i).data );
end

Sum21 = abs(Sum2) + 0.1;
SGN2 = Sum2./Sum21;

DT_i = -Observer_Gain1*epsilon_i - SGN2*diag(Upsilon_M);

end

== matlab function CAMFC2_Quad_New_02_Payload_01/Agent #3/Controller #3/Cooperative Observers #3/Observer q#3 ==
  data: q input; Dq_i output; tau input; H parameter; BN parameter; AN parameter; q_i input; u0 input; U_dot0_M parameter; tau_i output; N parameter; Agent_Num input; Observer_Gain parameter; n0 parameter; alpha parameter
function [Dq_i,tau_i] = fcn(q,tau,H,BN,AN,q_i,u0,U_dot0_M,N,Agent_Num,Observer_Gain,n0,alpha)

tau_i = + BN(Agent_Num,Agent_Num)*(q_i - u0);
Sum2 = zeros(n0,1);
for i=1:N
    tau_i = tau_i + ( AN(Agent_Num,i) * (q_i - q(((i-1)*n0+1):n0*i)) );  
    Sum2 = Sum2 + ( H(i,Agent_Num) * tau(((i-1)*n0+1):n0*i) );
end

Sum21 = abs(Sum2) + alpha;
SGN2 = Sum2./Sum21;

Dq_i = -Observer_Gain*tau_i - diag(SGN2)*U_dot0_M;

end

== matlab function CAMFC2_Quad_New_02_Payload_01/Agent #3/Controller #3/Cooperative Observers #3/Observer x0_hat#3 ==
  data: x0_hat input; Dx0_hat_i output; x0_tilde input; H parameter; BN parameter; AN parameter; x0_hat_i input; x0 input; X_M parameter; x0_tilde_i output; N parameter; Agent_Num input; Observer_Gain parameter; n0 parameter; alpha parameter
function [Dx0_hat_i,x0_tilde_i] = fcn(x0_hat,x0_tilde,H,BN,AN,x0_hat_i,x0,X_M,N,Agent_Num,Observer_Gain,n0,alpha)

x0_tilde_i = + BN(Agent_Num,Agent_Num)*(x0_hat_i - x0);
Sum2 = zeros(n0,1);
for i=1:N
    x0_tilde_i = x0_tilde_i + ( AN(Agent_Num,i) * (x0_hat_i - x0_hat(((i-1)*n0+1):n0*i)) );  
    Sum2 = Sum2 + ( H(i,Agent_Num) * x0_tilde(((i-1)*n0+1):n0*i) );
end

Sum21 = abs(Sum2) + alpha;
SGN2 = Sum2./Sum21;

Dx0_hat_i = -Observer_Gain*x0_tilde_i - diag(SGN2)*X_M;

end

== matlab function CAMFC2_Quad_New_02_Payload_01/Agent #3/Controller #3/Translational #3/Adaptive Law A_T #3 ==
  data: Agent_Num input; A_hat input; gama2 parameter; rho2 parameter; T_i input; P_i input; DA_hat output; e_i input; H parameter; BN parameter; N parameter; n parameter; n0 parameter; z0 input; x0_hat_inp input; ui input
function DA_hat = fcn(Agent_Num,A_hat,gama2,rho2,T_i,P_i,e_i,H,BN,N,n,n0,z0,x0_hat_inp,ui)

%% 
z0_i = [z0;ui(1:n0)]; 
x0_hat_i = [x0_hat_inp;ui(1:n0)];

%%
vA_hat = diag(A_hat);

Sum = zeros(n,1);
for i=2:(N+1)
    Sum = Sum + ( H(Agent_Num,(i-1)) * ( (2*x0_hat_i) - (2*[T_i(1,:)';zeros(n0,1)]) + ([T_i(i,:)';zeros(n0,1)]) ) );
end
Sum(1:n0) = Sum(1:n0) + ( BN(Agent_Num,Agent_Num)*z0_i(1:n0) ) - e_i(1:n0);
Sum(n0+1:n) = Sum(n0+1:n) + ( 1*z0_i(n0+1:n) ) - e_i(n0+1:n);
    
DvA_hat = -gama2*diag(Sum)*P_i * e_i - (rho2*gama2*vA_hat);

DA_hat = diag(DvA_hat);

end

== matlab function CAMFC2_Quad_New_02_Payload_01/Agent #3/Controller #3/Translational #3/Adaptive Law g_T #3 ==
  data: Agent_Num input; g_hat input; gama1 parameter; rho1 parameter; P input; P_struct parameter; Dg_hat output; e input; H parameter; N parameter; n parameter
function Dg_hat = fcn(Agent_Num,g_hat,gama1,rho1,P,P_struct,e,H,N,n)

P_struct(1).data = P.p1;
P_struct(2).data = P.p2;
P_struct(3).data = P.p3;
P_struct(4).data = P.p4;

Sum = zeros(n,1);
for i=1:N  
    Sum = Sum + (H(i,Agent_Num) * P_struct(i).data * e((i-1)*n+1:(i*n),1)); %Adaptive law
end
    
Dg_hat = -gama1*Sum - (rho1*gama1*g_hat);

end

== matlab function CAMFC2_Quad_New_02_Payload_01/Agent #3/Controller #3/Translational #3/DRE_T ==
  data: P input; A_hat input; B parameter; R parameter; DP output; Q parameter
function DP = fcn(P,A_hat,B,R,Q)

DP = 2*A_hat*P + 2*P*A_hat' - P*B*R*B'*P + 2*Q;

end

== matlab function CAMFC2_Quad_New_02_Payload_01/Agent #3/Controller #3/Translational #3/Differentiator1/Sliding differentiator ==
  data: u output; u1 input; e input; k1 parameter; alpha parameter
function u = fcn(u1,e,k1,alpha)

b=k1;

ABS = abs(e);
SGN = e ./ (ABS + alpha);
u = u1 - b*((ABS.^0.5).*SGN); 

end

== matlab function CAMFC2_Quad_New_02_Payload_01/Agent #4/Controller #4/Controller to Motors #4 ==
  data: u output; uT input; uR input; RM_1 parameter
function u = fcn(uT,uR,RM_1)

y1 = uR(4);
y2 = uR(5);
y3 = uR(6);

Y = [uT;y1;y2;y3];

u = RM_1*Y;

for i=1:4
    u(i) = sqrt(abs(u(i)));
end

end

== matlab function CAMFC2_Quad_New_02_Payload_01/Agent #3/Controller #3/Translational #3/Differentiator1/Sliding differentiator1 ==
  data: Du1 output; e input; k2 parameter; alpha parameter
function Du1 = fcn(e,k2,alpha)

a=k2;

ABS = abs(e);
SGN = e ./ (ABS + alpha);
Du1 = - a*SGN;

end

== matlab function CAMFC2_Quad_New_02_Payload_01/Agent #3/Plant #3/MATLAB Function ==
  data: X input; U input; t input; DX output; Kf parameter; Kt parameter; Kd parameter; Ka parameter; M parameter; J parameter; Lq parameter; ge parameter
function DX = fcn(X,U,t,Kf,Kt,Kd,Ka,M,J,Lq,ge)

phi = X(4);
theta = X(5);
psi = X(6);

Rq = [cos(psi)*cos(theta) -sin(psi)*cos(phi)+cos(psi)*sin(theta)*sin(phi) sin(psi)*sin(phi)+cos(psi)*sin(theta)*cos(phi);
    sin(psi)*cos(theta) cos(psi)*cos(phi)+sin(psi)*sin(theta)*sin(phi) -cos(psi)*sin(phi)+sin(psi)*sin(theta)*cos(phi);
    -sin(theta) cos(theta)*sin(phi) cos(theta)*cos(phi)]; 

R_omega = [1 0 -sin(theta);
    0 cos(phi) cos(theta)*sin(phi);
    0 -sin(phi) cos(theta)*cos(phi)];

EXT_PRD = External_Product3(X(10:12),(J*X(10:12)));

F1 = Kf * U(1)^2;
F2 = Kf * U(2)^2;
F3 = Kf * U(3)^2;
F4 = Kf * U(4)^2;
  
FT = F1 + F2 + F3 + F4;
 
T1 = Kt * U(1)^2;
T2 = Kt * U(2)^2;
T3 = Kt * U(3)^2;
T4 = Kt * U(4)^2;
 
TT1 = Lq*(F3-F1);
TT2 = Lq*(F4-F2);
TT3 = (T1-T2+T3-T4);

FTT = Rq * [0;0;FT];
FTx = FTT(1);
FTy = FTT(2);
FTz = FTT(3);

DP = X(7:9);
DPHI = (R_omega)^(-1) * X(10:12); 
Dv = (1/M)*([FTx;FTy;FTz] - Kd*X(7:9) - M*[0;0;ge]) + Rq*(0.1*sin(1*t))*[0;0;1]; 
Dw = (J^(-1))*([TT1;TT2;TT3] - Ka*X(10:12) - EXT_PRD) + (1*sin(1*t)*[1;1;1]);

DX = [DP;DPHI;Dv;Dw];

end

== matlab function CAMFC2_Quad_New_02_Payload_01/Agent #3/Controller #3/Translational #3/Main Controller_T #3 ==
  data: n parameter; n0 parameter; U output; R parameter; Q parameter; P_i input; e_i input; K parameter; Zeta_i input; BN parameter; A_hat_i input; u0 input; z0 input; DT_i input; T_i input; H parameter; q_i input; Agent_Num input; B_pseudo_inverse parameter; ui input; x0_hat_inp input; g_hat_i input; D_ui1 input
function U = fcn(n,n0,R,Q,P_i,e_i,K,Zeta_i,BN,A_hat_i,u0,z0,DT_i,T_i,H,q_i,Agent_Num,B_pseudo_inverse,ui,x0_hat_inp, g_hat_i, D_ui1)

D_eta_0 = [DT_i(1,:)';zeros(n0,1)];

%% 
z0_i = [z0;ui(1:n0)];
x0_hat_i = [x0_hat_inp;ui(1:n0)];
u0_i = [u0;D_ui1];

%%

S_H = sum(H(Agent_Num,:)) - H(Agent_Num,Agent_Num);
U4 = - S_H * ([q_i;u0_i(n0+1:n)] - [DT_i(1,:)';zeros(n0,1)] - (A_hat_i * (x0_hat_i - [T_i(1,:)';zeros(n0,1)])));
U1 = 1/2 * R * P_i * e_i; %Consensus Error
U5 = ( A_hat_i * ( H(Agent_Num,Agent_Num)*(2*x0_hat_i - 2*[T_i(1,:)';zeros(n0,1)] + [T_i(Agent_Num+1,:)';zeros(n0,1)]) ) ) - e_i;
U5(1:n0) = U5(1:n0) + ( BN(Agent_Num,Agent_Num) * z0_i(1:n0) );
U5(n0+1:n) = U5(n0+1:n) + ( 1 * z0_i(n0+1:n) );
U2 = - g_hat_i; %nonlinear compensation 
U3 = + [DT_i(Agent_Num+1,:)';zeros(n0,1)]; %Derivative of Formation parameters  
U6 = zeros(n,1);
U6(1:n0) = - BN(Agent_Num,Agent_Num)*( D_eta_0(1:n0) - u0_i(1:n0) ); %Connection to the leader
U6(n0+1:n) = - 1 * ( D_eta_0(n0+1:n) - u0_i(n0+1:n) );
U7 = K * Zeta_i; %Consensus time-integral
U8 = (2*Q - 3/4*R*P_i)*e_i;

U_input = U1 + U2 + U3 + U4 + U5 + U6 + U7 + U8;

U = B_pseudo_inverse * U_input / H(Agent_Num,Agent_Num);

end

== matlab function CAMFC2_Quad_New_02_Payload_01/Agent #3/Controller #3/Translational #3/Module to compute Consensus Error_T #3 ==
  data: T_i input; x input; x0 input; ep output; AN parameter; BN parameter; N parameter; n parameter; n0 parameter; Agent_Num input; ui input
function ep = fcn(T_i,x,x0,AN,BN,N,n,n0,Agent_Num,ui)

Diff_Star_to0 = (T_i((Agent_Num+1),:))';
Diff_Star_to_Other = (eye(n0) * Diff_Star_to0 * ones(1,N))' - T_i(2:N+1,:);
Diff_Star_to_Other = Diff_Star_to_Other';

xp = zeros(n,N);
for i=1:N
    xp(1:n,i) = [x((i-1)*(2*n)+1:(i-1)*(2*n)+n0);x((i-1)*(2*n)+(2*n0)+1:(i-1)*(2*n)+(2*n0)+n0)];
end

%%
xp_own = zeros(n,1);
xp_own(1:n,1) = xp(1:n,Agent_Num);

xp0 = [x0;ui(1:n0)];

xp_other = zeros(n,N);
ep = zeros(n,1);
ep(1:n0,1) = ep(1:n0,1) + ( BN(Agent_Num,Agent_Num)*(-(xp_own(1:n0)-xp0(1:n0))+Diff_Star_to0) );
ep(n0+1:n,1) = ep(n0+1:n,1) + ( 1*(-(xp_own(n0+1:n)-xp0(n0+1:n))) );

for i=1:N        
    xp_other(1:n,i) = xp(1:n,i);
    ep(1:n0,1) = ep(1:n0,1) + AN(Agent_Num,i)*(-(xp_own(1:n0)-xp_other(1:n0,i))+Diff_Star_to_Other(:,i));
    ep(n0+1:n,1) = ep(n0+1:n,1) + AN(Agent_Num,i)*(-(xp_own(n0+1:n)-xp_other(n0+1:n,i)));
end

end

== matlab function CAMFC2_Quad_New_02_Payload_01/Agent #4/Controller #4/Cooperative Observers #1/Differentiator2/Sliding differentiator ==
  data: u output; u1 input; e input; k1 parameter; alpha parameter
function u = fcn(u1,e,k1,alpha)

b=k1;

ABS = abs(e);
SGN = e ./ (ABS + alpha);
u = u1 - b*((ABS.^0.5).*SGN); 

end

== matlab function CAMFC2_Quad_New_02_Payload_01/Agent #4/Controller #4/Cooperative Observers #1/Differentiator2/Sliding differentiator1 ==
  data: Du1 output; e input; k2 parameter; alpha parameter
function Du1 = fcn(e,k2,alpha)

a=k2;

ABS = abs(e);
SGN = e ./ (ABS + alpha);
Du1 = - a*SGN;

end

== matlab function CAMFC2_Quad_New_02_Payload_01/Agent #4/Controller #4/Rotational/Differentiator/Sliding differentiator1 ==
  data: Du1 output; e input; n parameter; k2 parameter
function Du1 = fcn(e,n,k2)

a=k2;

ABS = zeros(n,1);
for i=1:n
    if e(i)>0
        ABS(i) = e(i);
    else
        ABS(i) = -e(i);
    end
end
SGN = e ./ (ABS + 0.01);

Du1 = - a*SGN;

end

== matlab function CAMFC2_Quad_New_02_Payload_01/Agent #4/Controller #4/Rotational/g-Estimator ==
  data: sigma input; g_hat input; P input; rho_1 parameter; gamma_1 parameter; Dg_hat output
function Dg_hat = fcn(sigma,g_hat,P,rho_1,gamma_1)

Dg_hat = - gamma_1 * P * sigma - rho_1 * gamma_1 * g_hat;

end
